simulink model "DePascali4M"  (R2015a)
settings: Solver=ode45  SolverMode=SingleTasking  StartTime=0.0  StopTime=15  RelTol=1e-5
values from neighbouring files (symbols this model uses):
  d1 = 500    [DePascali4Minit.m]    (also in M46Dinit.m)
  d2 = 500    [DePascali4Minit.m]    (also in M46Dinit.m)
  d3 = 500    [DePascali4Minit.m]    (also in M46Dinit.m)
  d4 = 500    [DePascali4Minit.m]    (also in M46Dinit.m)
  delta1 = 200    [DePascali4Minit.m]    (also in M46Dinit.m)
  delta2 = 200    [DePascali4Minit.m]    (also in M46Dinit.m)
  delta3 = 200    [DePascali4Minit.m]    (also in M46Dinit.m)
  delta4 = 200    [DePascali4Minit.m]    (also in M46Dinit.m)
  g = [0;0;9.81]    [DePascali4Minit.m]    (also in M46Dinit.m)
  j0 = 0.5    [DePascali4Minit.m]    (also in M46Dinit.m)
  j1 = 10    [DePascali4Minit.m]    (also in M46Dinit.m = 1)
  j1d = j1    (= 10)    [DePascali4Minit.m]
  j2 = 10    [DePascali4Minit.m]    (also in M46Dinit.m = 1)
  j2d = j2    (= 10)    [DePascali4Minit.m]
  j3 = 10    [DePascali4Minit.m]    (also in M46Dinit.m = 1)
  j3d = j3    (= 10)    [DePascali4Minit.m]
  j4d = j4    (= 10)    [DePascali4Minit.m]
  k1 = 50    [DePascali4Minit.m]    (also in M46Dinit.m = 100)
  k2 = 50    [DePascali4Minit.m]    (also in M46Dinit.m = 100)
  k3 = 50    [DePascali4Minit.m]    (also in M46Dinit.m = 100)
  k4 = 50    [DePascali4Minit.m]    (also in M46Dinit.m = 100)
  kappa1 = 10    [DePascali4Minit.m]    (also in M46Dinit.m = 100)
  kappa2 = 10    [DePascali4Minit.m]    (also in M46Dinit.m = 100)
  kappa3 = 10    [DePascali4Minit.m]    (also in M46Dinit.m = 100)
  kappa4 = 10    [DePascali4Minit.m]    (also in M46Dinit.m = 100)
  m0 = 20    [DePascali4Minit.m]    (also in M46Dinit.m)
  m1 = 100    [DePascali4Minit.m]    (also in M46Dinit.m = 10)
  m1d = m1    (= 100)    [DePascali4Minit.m]
  m2 = 100    [DePascali4Minit.m]    (also in M46Dinit.m = 10)
  m2d = m2    (= 100)    [DePascali4Minit.m]
  m3 = 100    [DePascali4Minit.m]    (also in M46Dinit.m = 10)
  m3d = m3    (= 100)    [DePascali4Minit.m]
  m4 = 100    [DePascali4Minit.m]    (also in M46Dinit.m = 10)
  m4d = m4    (= 100)    [DePascali4Minit.m]
libraries: aerolibutil x7, dspinverses x1
settings Model: CovSFcnEnable=off  Creator=Martin  LastModifiedBy=mangerer
settings DataIOCC: LimitDataPoints=off
settings OptimizationCC: BlockReduction=off  BooleanDataType=off
settings DebuggingCC: SaveWithParameterizedLinksMsg=none  UnderspecifiedInitializationDetection=Classic  MergeDetectMultiDrivingBlocksExec=none  SignalResolutionControl=TryResolveAllWithWarning
settings HardwareCC: TargetUnknown=on

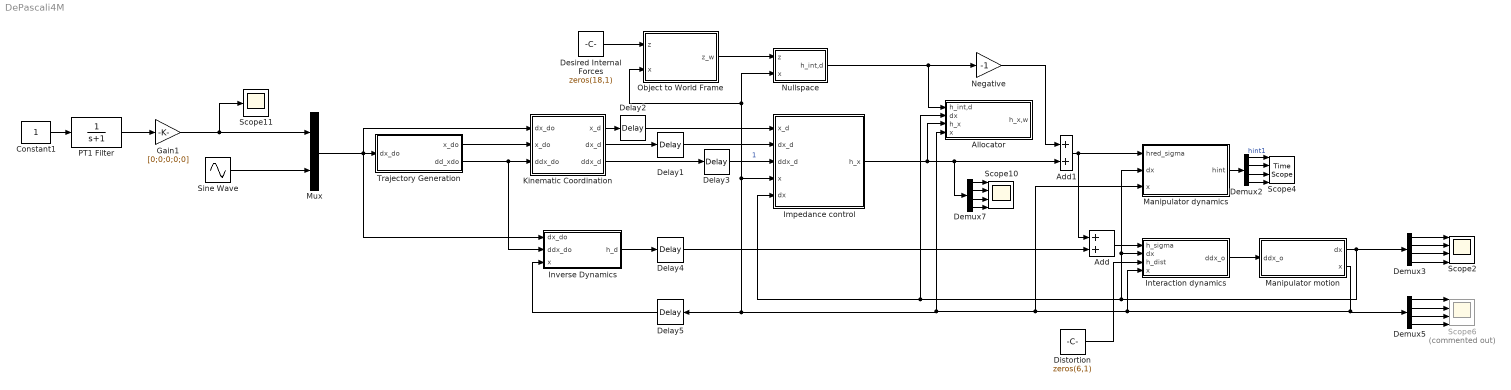
== system DePascali4M ==
  Add : Sum
  Add1 : Sum
  Allocator : Subsystem
  Constant1 : Constant
  Delay1 : TransportDelay  DelayTime=0
  Delay2 : TransportDelay  DelayTime=0  InitialOutput="[1 0 0 1 0 0 0   0 1 0 1 0 0 0    -1 0 0 1 0 0 0     0 -1 0 1 0 0 0]'"
  Delay3 : TransportDelay  DelayTime=0
  Delay4 : TransportDelay  DelayTime=0
  Delay5 : TransportDelay  DelayTime=0  InitialOutput="[1 0 0 1 0 0 0   0 1 0 1 0 0 0    -1 0 0 1 0 0 0     0 -1 0 1 0 0 0]'"
  Demux{2..3,5,7} (4 alike) : Demux
  Desired Internal Forces : Constant  Value=zeros(18,1)
  Distortion : Constant  Value=zeros(6,1)
  Gain1 : Gain  Gain=[0;0;0;0;0]
  Impedance control : Subsystem
  Interaction dynamics : Subsystem
  Inverse Dynamics : Subsystem
  Kinematic Coordination : Subsystem
  Manipulator dynamics : Subsystem
  Manipulator motion : Subsystem
  Mux : Mux  Inputs=2
  Negative : Gain  Gain=-1
  Nullspace : Subsystem
  Object to World Frame : MATLAB Function  TreatAsAtomicUnit=on
  PT1 Filter : TransferFcn  Denominator=[1 1]
  Scope10 : Scope  NumInputPorts=4
      settings: ShowLegends=on  YMin=-1~-5~-5~-5  YMax=1~5~5~5  SaveName=ScopeData18
  Scope11 : Scope
      settings: YMin=0.9984  YMax=1  SaveName=ScopeData26
  Scope2 : Scope  NumInputPorts=4
      settings: ShowLegends=on  YMin=-1.5~-1.5~-1.5~-1.5  YMax=6~5.5~6~5.5  SaveName=ScopeData2
  Scope4 : TimeScope  NumInputPorts=4
  Scope6 : Scope  Commented=on  NumInputPorts=4
      settings: ShowLegends=on  YMin=-25~-25~-25~-25  YMax=200~200~200~200  SaveName=ScopeData11
  Sine Wave : Sin  Frequency=2*pi  SampleTime=0
  Trajectory Generation : Subsystem
  wires:
  Interaction dynamics/1(ddx_o) -> Manipulator motion/1(ddx_o)
  Manipulator dynamics/1(hint) -> Demux2/1
  Demux2/1 -> Scope4/1  "hint1"
  Demux2/2 -> Scope4/2
  Demux2/3 -> Scope4/3
  Demux2/4 -> Scope4/4
  Demux3/1 -> Scope2/1
  Demux3/2 -> Scope2/2
  Demux3/3 -> Scope2/3
  Demux3/4 -> Scope2/4
  Add1/1 -> Manipulator dynamics/1(hred_sigma), Add/1
  Demux5/1 -> Scope6/1
  Demux5/2 -> Scope6/2
  Demux5/3 -> Scope6/3
  Demux5/4 -> Scope6/4
  Object to World Frame/1(z_w) -> Nullspace/1(z)
  Nullspace/1(h_int,d) -> Negative/1, Allocator/1(h_int,d)
  Desired Internal Forces/1 -> Object to World Frame/1(z)
  Demux7/1 -> Scope10/1
  Demux7/2 -> Scope10/2
  Demux7/3 -> Scope10/3
  Demux7/4 -> Scope10/4
  PT1 Filter/1 -> Gain1/1
  Add/1 -> Interaction dynamics/1(h_sigma)
  Gain1/1 -> Scope11/1, Mux/1
  Impedance control/1(h_x) -> Demux7/1, Add1/2, Allocator/3(h_x)
  Manipulator motion/1(dx) -> Demux3/1, Impedance control/5(dx), Allocator/2(dx), Interaction dynamics/2(dx), Manipulator dynamics/2(dx)
  Inverse Dynamics/1(h_d) -> Delay4/1
  Sine Wave/1 -> Mux/2
  Kinematic Coordination/1(x_d) -> Delay2/1
  Kinematic Coordination/2(dx_d) -> Delay1/1
  Kinematic Coordination/3(ddx_d) -> Delay3/1
  Trajectory Generation/2(dd_xdo) -> Kinematic Coordination/3(ddx_do), Inverse Dynamics/2(ddx_do)
  Trajectory Generation/1(x_do) -> Kinematic Coordination/2(x_do)
  Mux/1 -> Kinematic Coordination/1(dx_do), Inverse Dynamics/1(dx_do), Trajectory Generation/1(dx_do)
  Delay2/1 -> Impedance control/1(x_d)
  Delay1/1 -> Impedance control/2(dx_d)
  Delay3/1 -> Impedance control/3(ddx_d)  "1"
  Delay4/1 -> Add/2
  Manipulator motion/2(x) -> Demux5/1, Interaction dynamics/4(x), Manipulator dynamics/3(x), Impedance control/4(x), Object to World Frame/2(x), Nullspace/2(x), Delay5/1, Allocator/4(x)
  Delay5/1 -> Inverse Dynamics/3(x)
  Negative/1 -> Add1/1
  Constant1/1 -> PT1 Filter/1
  Distortion/1 -> Interaction dynamics/3(h_dist)

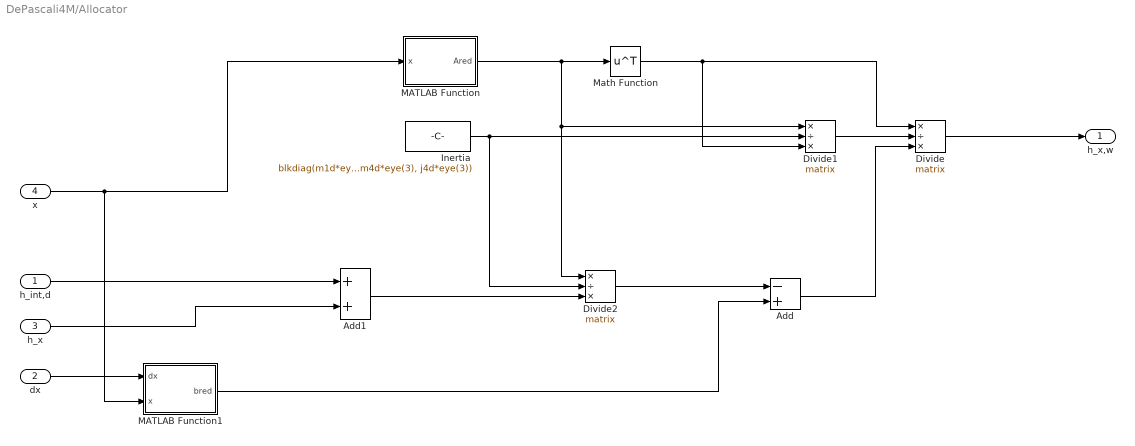
== system DePascali4M/Allocator ==
  h_int,d : Inport
  dx : Inport  Port=2
  h_x : Inport  Port=3
  x : Inport  Port=4
  Add : Sum  Inputs=-+
  Add1 : Sum
  Divide : Product  Inputs=*/*  Multiplication=Matrix(*)
  Divide1 : Product  Inputs=*/*  Multiplication=Matrix(*)
  Divide2 : Product  Inputs=*/*  Multiplication=Matrix(*)
  Inertia : Constant  Value=blkdiag(m1d*eye(3), j1d*eye(3), m2d*eye(3), j2d*eye(3), m3d*eye(3), j3d*eye(3), m4d*eye(3), j4d*eye(3))
  MATLAB Function : MATLAB Function  TreatAsAtomicUnit=on
  MATLAB Function1 : MATLAB Function  TreatAsAtomicUnit=on
  Math Function : Math  Operator=transpose  SaturateOnIntegerOverflow=on
  h_x,w : Outport
  wires:
  dx/1 -> MATLAB Function1/1(dx)
  Divide/1 -> h_x,w/1
  Math Function/1 -> Divide1/3, Divide/1
  MATLAB Function/1(Ared) -> Math Function/1, Divide2/1, Divide1/1
  Divide1/1 -> Divide/2
  Inertia/1 -> Divide1/2, Divide2/2
  MATLAB Function1/1(bred) -> Add/2
  Add/1 -> Divide/3
  Divide2/1 -> Add/1
  Add1/1 -> Divide2/3
  h_int,d/1 -> Add1/1
  h_x/1 -> Add1/2
  x/1 -> MATLAB Function1/2(x), MATLAB Function/1(x)

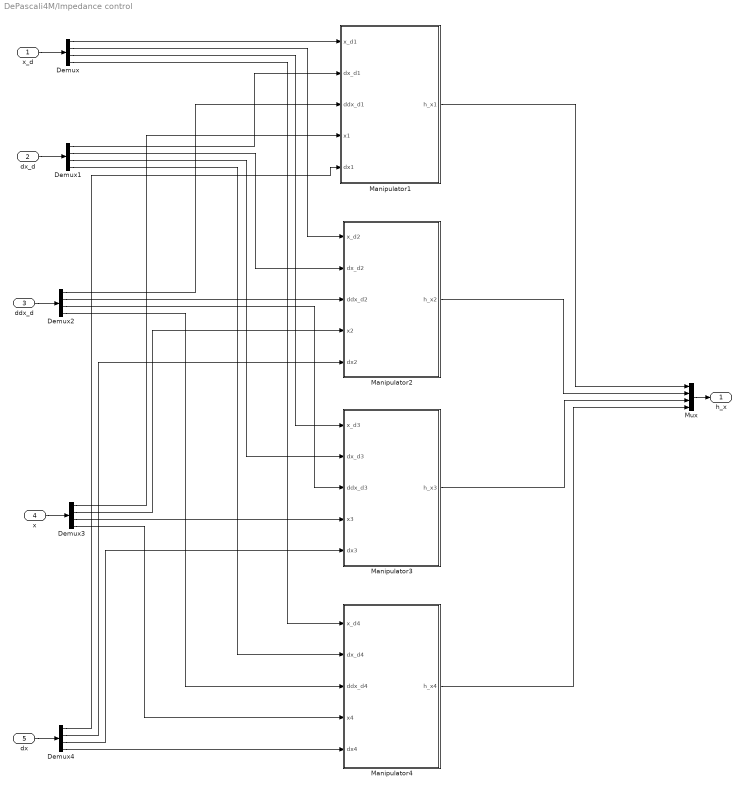
== system DePascali4M/Impedance control ==
  x_d : Inport
  dx_d : Inport  Port=2
  ddx_d : Inport  Port=3
  x : Inport  Port=4
  dx : Inport  Port=5
  Demux{,1..4} (5 alike) : Demux
  Manipulator1 : Subsystem
  Manipulator2 : Subsystem
  Manipulator3 : Subsystem
  Manipulator4 : Subsystem
  Mux : Mux
  h_x : Outport
  wires:
  dx/1 -> Demux4/1
  x/1 -> Demux3/1
  ddx_d/1 -> Demux2/1
  dx_d/1 -> Demux1/1
  x_d/1 -> Demux/1
  Demux/1 -> Manipulator1/1(x_d1)
  Demux/2 -> Manipulator2/1(x_d2)
  Demux/3 -> Manipulator3/1(x_d3)
  Demux/4 -> Manipulator4/1(x_d4)
  Demux1/1 -> Manipulator1/2(dx_d1)
  Demux1/2 -> Manipulator2/2(dx_d2)
  Demux1/3 -> Manipulator3/2(dx_d3)
  Demux1/4 -> Manipulator4/2(dx_d4)
  Demux2/1 -> Manipulator1/3(ddx_d1)
  Demux2/2 -> Manipulator2/3(ddx_d2)
  Demux2/3 -> Manipulator3/3(ddx_d3)
  Demux2/4 -> Manipulator4/3(ddx_d4)
  Demux3/1 -> Manipulator1/4(x1)
  Demux3/2 -> Manipulator2/4(x2)
  Demux3/3 -> Manipulator3/4(x3)
  Demux3/4 -> Manipulator4/4(x4)
  Demux4/4 -> Manipulator4/5(dx4)
  Demux4/3 -> Manipulator3/5(dx3)
  Demux4/2 -> Manipulator2/5(dx2)
  Demux4/1 -> Manipulator1/5(dx1)
  Mux/1 -> h_x/1
  Manipulator1/1(h_x1) -> Mux/1
  Manipulator2/1(h_x2) -> Mux/2
  Manipulator3/1(h_x3) -> Mux/3
  Manipulator4/1(h_x4) -> Mux/4

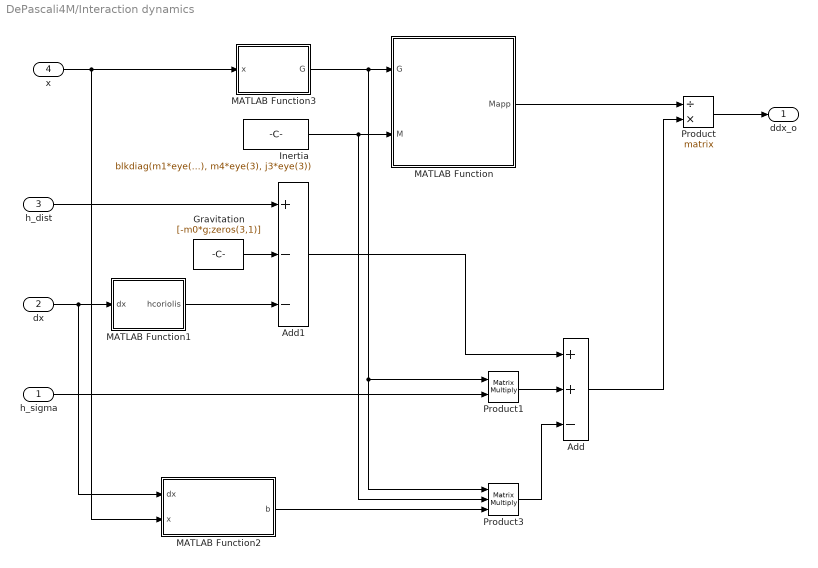
== system DePascali4M/Interaction dynamics ==
  h_sigma : Inport
  dx : Inport  Port=2
  h_dist : Inport  Port=3
  x : Inport  Port=4
  Add : Sum  Inputs=++-
  Add1 : Sum  Inputs=+--
  Gravitation : Constant  Value=[-m0*g;zeros(3,1)]
  Inertia : Constant  Value=blkdiag(m1*eye(3), j1*eye(3), m2*eye(3), j2*eye(3), m3*eye(3), j3*eye(3), m4*eye(3), j3*eye(3))
  MATLAB Function : MATLAB Function  TreatAsAtomicUnit=on
  MATLAB Function1 : MATLAB Function  TreatAsAtomicUnit=on
  MATLAB Function2 : MATLAB Function  TreatAsAtomicUnit=on
  MATLAB Function3 : MATLAB Function  TreatAsAtomicUnit=on
  Product : Product  Inputs=/*  Multiplication=Matrix(*)
  Product1 : Product  Multiplication=Matrix(*)
  Product3 : Product  Inputs=***  Multiplication=Matrix(*)
  ddx_o : Outport
  wires:
  MATLAB Function3/1(G) -> Product1/1, Product3/1, MATLAB Function/1(G)
  Inertia/1 -> Product3/2, MATLAB Function/2(M)
  MATLAB Function/1(Mapp) -> Product/1
  Add/1 -> Product/2
  Product1/1 -> Add/2
  h_sigma/1 -> Product1/2
  Add1/1 -> Add/1
  h_dist/1 -> Add1/1
  Gravitation/1 -> Add1/2
  dx/1 -> MATLAB Function2/1(dx), MATLAB Function1/1(dx)
  MATLAB Function1/1(hcoriolis) -> Add1/3
  Product3/1 -> Add/3
  MATLAB Function2/1(b) -> Product3/3
  Product/1 -> ddx_o/1
  x/1 -> MATLAB Function2/2(x), MATLAB Function3/1(x)

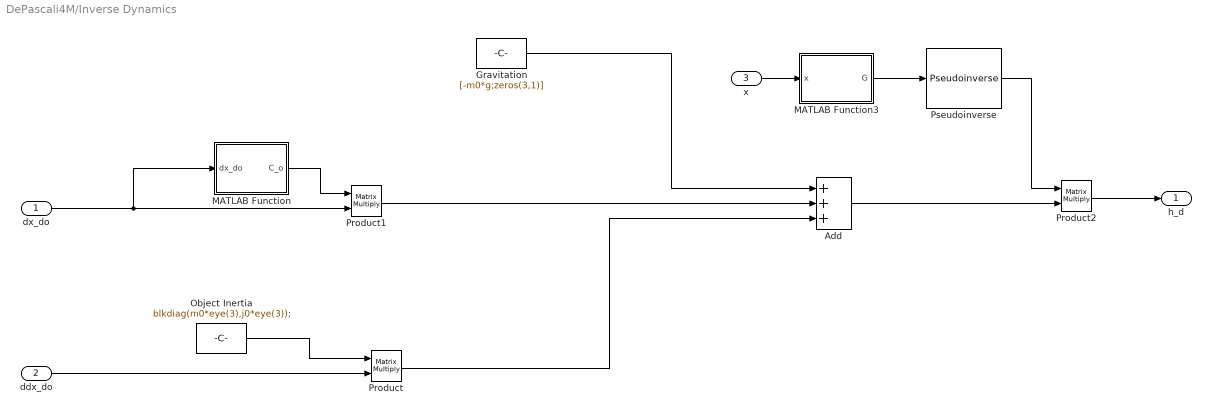
== system DePascali4M/Inverse Dynamics ==
  dx_do : Inport
  ddx_do : Inport  Port=2
  x : Inport  Port=3
  Add : Sum  Inputs=+++
  Gravitation : Constant  Value=[-m0*g;zeros(3,1)]
  MATLAB Function : MATLAB Function  TreatAsAtomicUnit=on
  MATLAB Function3 : MATLAB Function  TreatAsAtomicUnit=on
  Object Inertia : Constant  Value=blkdiag(m0*eye(3),j0*eye(3));
  Product : Product  Multiplication=Matrix(*)
  Product1 : Product  Multiplication=Matrix(*)
  Product2 : Product  Multiplication=Matrix(*)
  Pseudoinverse : dspinverses/Pseudoinverse  wanterr=off
  h_d : Outport
  wires:
  ddx_do/1 -> Product/2
  Object Inertia/1 -> Product/1
  dx_do/1 -> Product1/2, MATLAB Function/1(dx_do)
  MATLAB Function/1(C_o) -> Product1/1
  Product1/1 -> Add/2
  Gravitation/1 -> Add/1
  MATLAB Function3/1(G) -> Pseudoinverse/1
  Pseudoinverse/1 -> Product2/1
  Product2/1 -> h_d/1
  x/1 -> MATLAB Function3/1(x)
  Product/1 -> Add/3
  Add/1 -> Product2/2

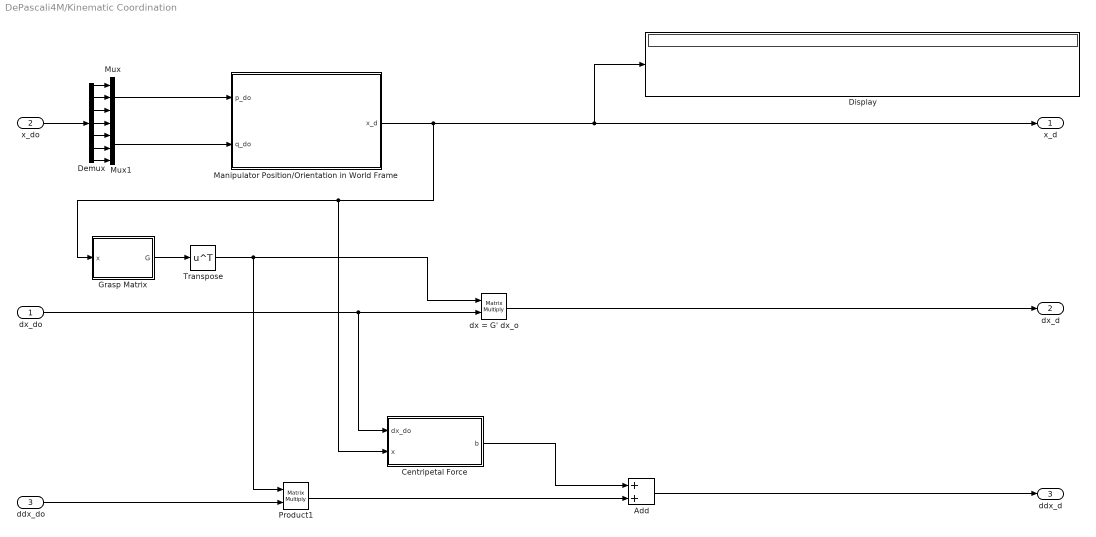
== system DePascali4M/Kinematic Coordination ==
  dx_do : Inport
  x_do : Inport  Port=2
  ddx_do : Inport  Port=3
  Add : Sum
  Centripetal Force : MATLAB Function  TreatAsAtomicUnit=on
  Demux : Demux  Outputs=7
  Display : Display
  Grasp Matrix : MATLAB Function  TreatAsAtomicUnit=on
  Manipulator Position/Orientation in World Frame : MATLAB Function  TreatAsAtomicUnit=on
  Mux : Mux  Inputs=3
  Mux1 : Mux
  Product1 : Product  Multiplication=Matrix(*)
  Transpose : Math  Operator=transpose  SaturateOnIntegerOverflow=on
  dx = G' dx_o : Product  Multiplication=Matrix(*)
  x_d : Outport
  dx_d : Outport  Port=2
  ddx_d : Outport  Port=3
  wires:
  Grasp Matrix/1(G) -> Transpose/1
  Transpose/1 -> Product1/1, dx = G' dx_o/1
  dx_do/1 -> Centripetal Force/1(dx_do), dx = G' dx_o/2
  dx = G' dx_o/1 -> dx_d/1
  x_do/1 -> Demux/1
  Demux/1 -> Mux/1
  Demux/2 -> Mux/2
  Demux/3 -> Mux/3
  Demux/5 -> Mux1/2
  Demux/6 -> Mux1/3
  Demux/7 -> Mux1/4
  Demux/4 -> Mux1/1
  Mux1/1 -> Manipulator Position/Orientation in World Frame/2(q_do)
  Mux/1 -> Manipulator Position/Orientation in World Frame/1(p_do)
  Centripetal Force/1(b) -> Add/1
  ddx_do/1 -> Product1/2
  Product1/1 -> Add/2
  Add/1 -> ddx_d/1
  Manipulator Position/Orientation in World Frame/1(x_d) -> Centripetal Force/2(x), Grasp Matrix/1(x), Display/1, x_d/1

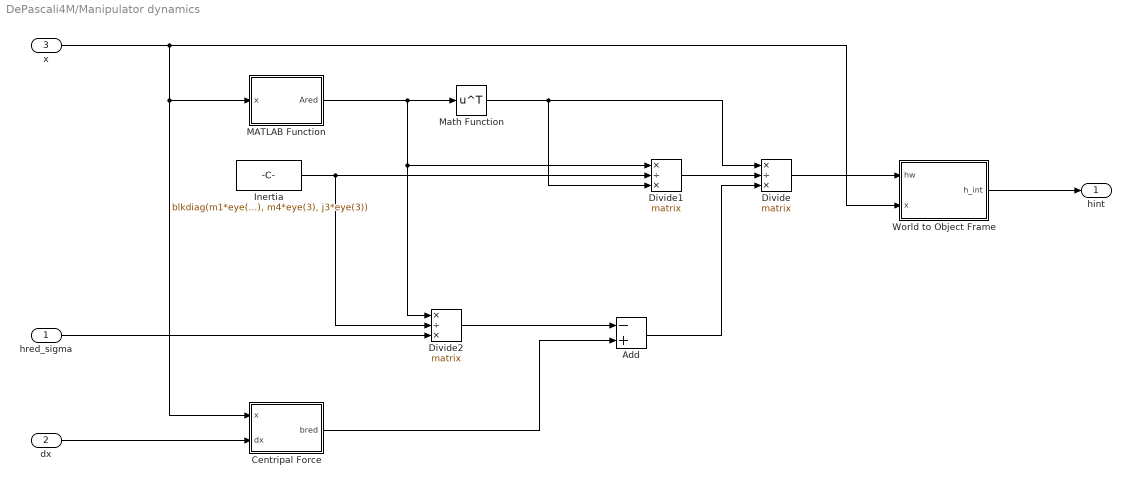
== system DePascali4M/Manipulator dynamics ==
  hred_sigma : Inport
  dx : Inport  Port=2
  x : Inport  Port=3
  Add : Sum  Inputs=-+
  Centripal Force : MATLAB Function  TreatAsAtomicUnit=on
  Divide : Product  Inputs=*/*  Multiplication=Matrix(*)
  Divide1 : Product  Inputs=*/*  Multiplication=Matrix(*)
  Divide2 : Product  Inputs=*/*  Multiplication=Matrix(*)
  Inertia : Constant  Value=blkdiag(m1*eye(3), j1*eye(3), m2*eye(3), j2*eye(3), m3*eye(3), j3*eye(3), m4*eye(3), j3*eye(3))
  MATLAB Function : MATLAB Function  TreatAsAtomicUnit=on
  Math Function : Math  Operator=transpose  SaturateOnIntegerOverflow=on
  World to Object Frame : MATLAB Function  TreatAsAtomicUnit=on
  hint : Outport
  wires:
  Math Function/1 -> Divide1/3, Divide/1
  MATLAB Function/1(Ared) -> Math Function/1, Divide2/1, Divide1/1
  Divide1/1 -> Divide/2
  Inertia/1 -> Divide1/2, Divide2/2
  dx/1 -> Centripal Force/2(dx)
  Add/1 -> Divide/3
  Divide2/1 -> Add/1
  hred_sigma/1 -> Divide2/3
  Divide/1 -> World to Object Frame/1(hw)
  World to Object Frame/1(h_int) -> hint/1
  x/1 -> Centripal Force/1(x), MATLAB Function/1(x), World to Object Frame/2(x)
  Centripal Force/1(bred) -> Add/2

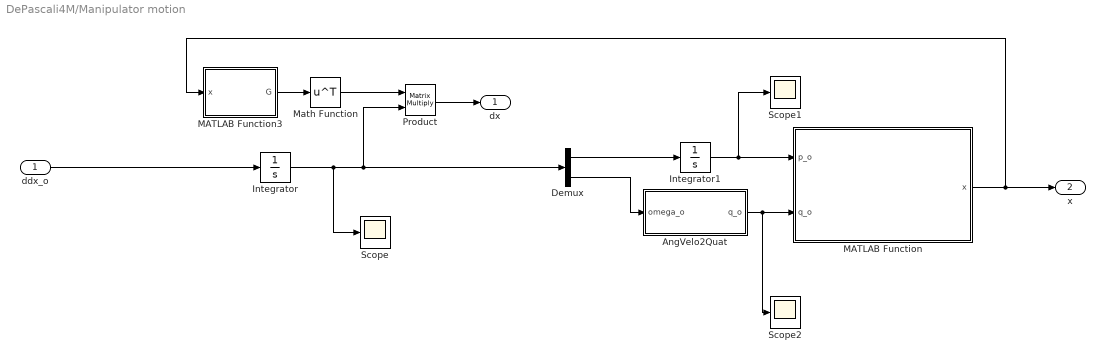
== system DePascali4M/Manipulator motion ==
  ddx_o : Inport
  AngVelo2Quat : Subsystem
  Demux : Demux  Outputs=2
  Integrator : Integrator  InitialCondition=zeros(6,1)
  Integrator1 : Integrator  InitialCondition=[0 0 0]'
  MATLAB Function : MATLAB Function  TreatAsAtomicUnit=on
  MATLAB Function3 : MATLAB Function  TreatAsAtomicUnit=on
  Math Function : Math  Operator=transpose  SaturateOnIntegerOverflow=on
  Product : Product  Multiplication=Matrix(*)
  Scope : Scope
      settings: SaveName=ScopeData14
  Scope1 : Scope
      settings: SaveName=ScopeData15
  Scope2 : Scope
      settings: SaveName=ScopeData23
  dx : Outport
  x : Outport  Port=2
  wires:
  ddx_o/1 -> Integrator/1
  Integrator/1 -> Scope/1, Product/2, Demux/1
  MATLAB Function3/1(G) -> Math Function/1
  Math Function/1 -> Product/1
  Product/1 -> dx/1
  Demux/2 -> AngVelo2Quat/1(omega_o)
  Demux/1 -> Integrator1/1
  AngVelo2Quat/1(q_o) -> Scope2/1, MATLAB Function/2(q_o)
  Integrator1/1 -> Scope1/1, MATLAB Function/1(p_o)
  MATLAB Function/1(x) -> MATLAB Function3/1(x), x/1

== system DePascali4M/Nullspace ==
  z : Inport
  x : Inport  Port=2
  MATLAB Function : MATLAB Function  TreatAsAtomicUnit=on
  Math Function : Math  Operator=transpose  SaturateOnIntegerOverflow=on
  Product : Product  Multiplication=Matrix(*)
  h_int,d : Outport
  wires:
  MATLAB Function/1(Ared) -> Math Function/1
  Math Function/1 -> Product/1
  z/1 -> Product/2
  Product/1 -> h_int,d/1
  x/1 -> MATLAB Function/1(x)

== system DePascali4M/Trajectory Generation ==
  dx_do : Inport
  Angular Velocity to Quaternion Orientation : Subsystem
  Demux : Demux  Outputs=2
  Derivative : Derivative
  Integrator : Integrator  InitialCondition=zeros(3,1)
  Mux : Mux  Inputs=2
  Scope : Scope
      settings: YMin=-12.5  YMax=12.5  SaveName=ScopeData25
  x_do : Outport
  dd_xdo : Outport  Port=2
  wires:
  dx_do/1 -> Derivative/1, Demux/1
  Demux/2 -> Angular Velocity to Quaternion Orientation/1(omega_do)
  Demux/1 -> Integrator/1
  Angular Velocity to Quaternion Orientation/1(q_do) -> Mux/2
  Integrator/1 -> Mux/1
  Mux/1 -> x_do/1
  Derivative/1 -> Scope/1, dd_xdo/1

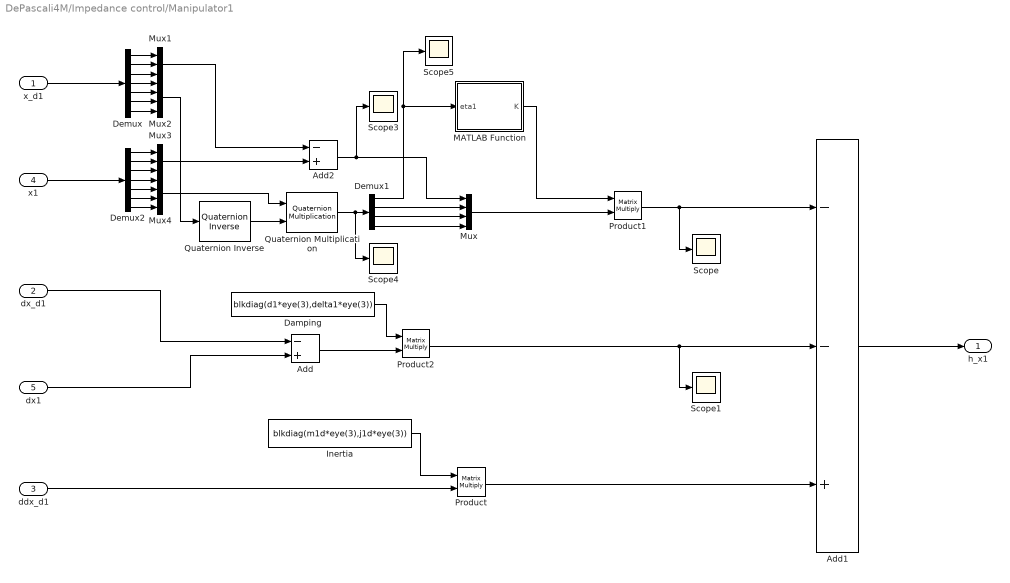
== system DePascali4M/Impedance control/Manipulator1 ==
  x_d1 : Inport
  dx_d1 : Inport  Port=2
  ddx_d1 : Inport  Port=3
  x1 : Inport  Port=4
  dx1 : Inport  Port=5
  Add : Sum  Inputs=-+
  Add1 : Sum  Inputs=--+
  Add2 : Sum  Inputs=-+
  Damping : Constant  Value=blkdiag(d1*eye(3),delta1*eye(3))
  Demux : Demux  Outputs=7
  Demux1 : Demux
  Demux2 : Demux  Outputs=7
  Inertia : Constant  Value=blkdiag(m1d*eye(3),j1d*eye(3))
  MATLAB Function : MATLAB Function  TreatAsAtomicUnit=on
  Mux : Mux
  Mux1 : Mux  Inputs=3
  Mux2 : Mux
  Mux3 : Mux  Inputs=3
  Mux4 : Mux
  Product : Product  Multiplication=Matrix(*)
  Product1 : Product  Multiplication=Matrix(*)
  Product2 : Product  Multiplication=Matrix(*)
  Quaternion Inverse : aerolibutil/Quaternion Inverse
  Quaternion Multiplication : aerolibutil/Quaternion Multiplication
  Scope{,1,3..5} (5 alike) : Scope
      Scope settings: TimeRange=200  YMin=-50  YMax=125  SaveName=ScopeData13
      Scope1 settings: TimeRange=200  YMin=-50  YMax=125  SaveName=ScopeData19
      Scope3 settings: ShowLegends=on  TimeRange=200  YMin=-50  YMax=125  SaveName=ScopeData21
      Scope4 settings: ShowLegends=on  TimeRange=50  YMin=-0.05  YMax=1  SaveName=ScopeData22
      Scope5 settings: ShowLegends=on  TimeRange=200  YMin=-50  YMax=125  SaveName=ScopeData24
  h_x1 : Outport
  wires:
  Add/1 -> Product2/2
  Damping/1 -> Product2/1
  dx_d1/1 -> Add/1
  dx1/1 -> Add/2
  MATLAB Function/1(K) -> Product1/1
  Demux1/1 -> MATLAB Function/1(eta1), Scope5/1
  Add2/1 -> Scope3/1, Mux/1
  Demux1/2 -> Mux/2
  Demux1/3 -> Mux/3
  Demux1/4 -> Mux/4
  x1/1 -> Demux2/1
  x_d1/1 -> Demux/1
  Demux/2 -> Mux1/2
  Demux/1 -> Mux1/1
  Demux/3 -> Mux1/3
  Demux/4 -> Mux2/1
  Demux/5 -> Mux2/2
  Demux/6 -> Mux2/3
  Demux/7 -> Mux2/4
  Demux2/2 -> Mux3/2
  Demux2/1 -> Mux3/1
  Demux2/3 -> Mux3/3
  Demux2/4 -> Mux4/1
  Demux2/5 -> Mux4/2
  Demux2/6 -> Mux4/3
  Demux2/7 -> Mux4/4
  Mux1/1 -> Add2/1
  Mux3/1 -> Add2/2
  Quaternion Multiplication/1 -> Scope4/1, Demux1/1
  Mux/1 -> Product1/2
  Inertia/1 -> Product/1
  Add1/1 -> h_x1/1
  Product1/1 -> Scope/1, Add1/1
  Product2/1 -> Scope1/1, Add1/2
  Product/1 -> Add1/3
  Quaternion Inverse/1 -> Quaternion Multiplication/2
  Mux4/1 -> Quaternion Multiplication/1
  Mux2/1 -> Quaternion Inverse/1
  ddx_d1/1 -> Product/2

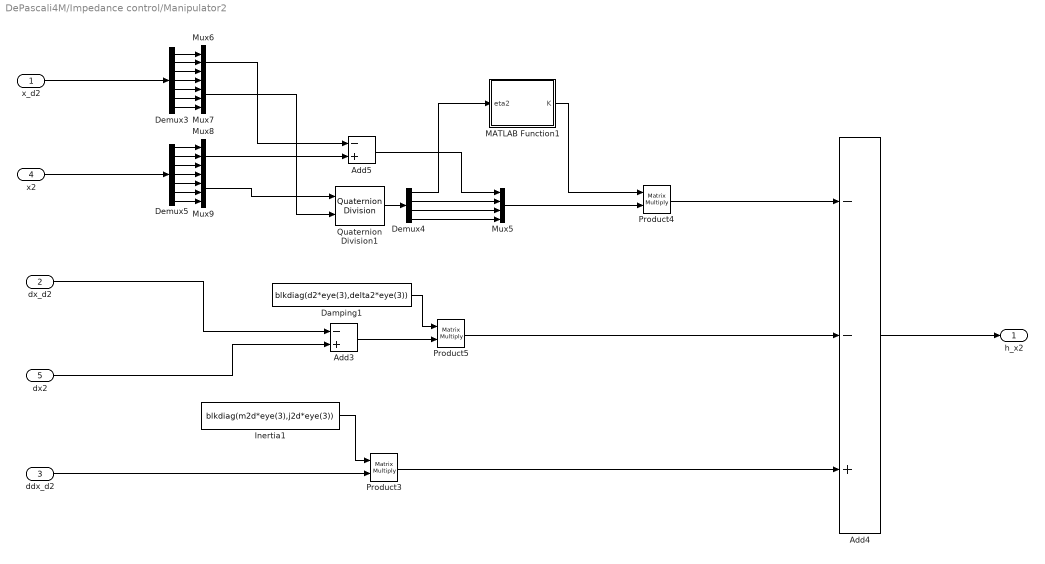
== system DePascali4M/Impedance control/Manipulator2 ==
  x_d2 : Inport
  dx_d2 : Inport  Port=2
  ddx_d2 : Inport  Port=3
  x2 : Inport  Port=4
  dx2 : Inport  Port=5
  Add3 : Sum  Inputs=-+
  Add4 : Sum  Inputs=--+
  Add5 : Sum  Inputs=-+
  Damping1 : Constant  Value=blkdiag(d2*eye(3),delta2*eye(3))
  Demux3 : Demux  Outputs=7
  Demux4 : Demux
  Demux5 : Demux  Outputs=7
  Inertia1 : Constant  Value=blkdiag(m2d*eye(3),j2d*eye(3))
  MATLAB Function1 : MATLAB Function  TreatAsAtomicUnit=on
  Mux5 : Mux
  Mux6 : Mux  Inputs=3
  Mux7 : Mux
  Mux8 : Mux  Inputs=3
  Mux9 : Mux
  Product3 : Product  Multiplication=Matrix(*)
  Product4 : Product  Multiplication=Matrix(*)
  Product5 : Product  Multiplication=Matrix(*)
  Quaternion Division1 : aerolibutil/Quaternion Division
  h_x2 : Outport
  wires:
  Add3/1 -> Product5/2
  Damping1/1 -> Product5/1
  dx_d2/1 -> Add3/1
  dx2/1 -> Add3/2
  MATLAB Function1/1(K) -> Product4/1
  Demux4/1 -> MATLAB Function1/1(eta2)
  Add5/1 -> Mux5/1
  Demux4/2 -> Mux5/2
  Demux4/3 -> Mux5/3
  Demux4/4 -> Mux5/4
  x2/1 -> Demux5/1
  x_d2/1 -> Demux3/1
  Demux3/2 -> Mux6/2
  Demux3/1 -> Mux6/1
  Demux3/3 -> Mux6/3
  Demux3/4 -> Mux7/1
  Demux3/5 -> Mux7/2
  Demux3/6 -> Mux7/3
  Demux3/7 -> Mux7/4
  Demux5/2 -> Mux8/2
  Demux5/1 -> Mux8/1
  Demux5/3 -> Mux8/3
  Demux5/4 -> Mux9/1
  Demux5/5 -> Mux9/2
  Demux5/6 -> Mux9/3
  Demux5/7 -> Mux9/4
  Mux6/1 -> Add5/1
  Mux8/1 -> Add5/2
  Quaternion Division1/1 -> Demux4/1
  Mux5/1 -> Product4/2
  Inertia1/1 -> Product3/1
  Add4/1 -> h_x2/1
  Product4/1 -> Add4/1
  Product5/1 -> Add4/2
  Product3/1 -> Add4/3
  Mux7/1 -> Quaternion Division1/2
  Mux9/1 -> Quaternion Division1/1
  ddx_d2/1 -> Product3/2

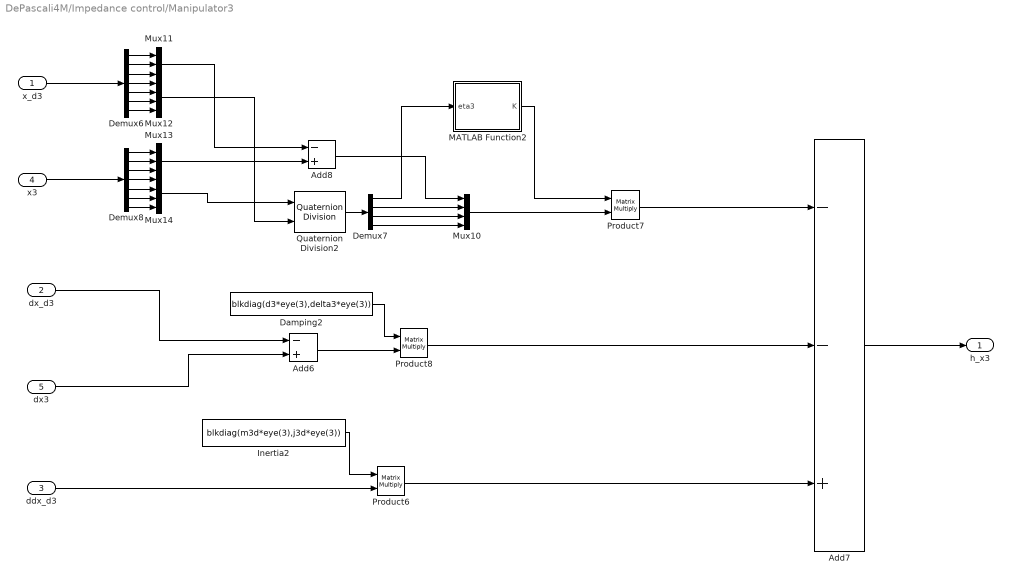
== system DePascali4M/Impedance control/Manipulator3 ==
  x_d3 : Inport
  dx_d3 : Inport  Port=2
  ddx_d3 : Inport  Port=3
  x3 : Inport  Port=4
  dx3 : Inport  Port=5
  Add6 : Sum  Inputs=-+
  Add7 : Sum  Inputs=--+
  Add8 : Sum  Inputs=-+
  Damping2 : Constant  Value=blkdiag(d3*eye(3),delta3*eye(3))
  Demux6 : Demux  Outputs=7
  Demux7 : Demux
  Demux8 : Demux  Outputs=7
  Inertia2 : Constant  Value=blkdiag(m3d*eye(3),j3d*eye(3))
  MATLAB Function2 : MATLAB Function  TreatAsAtomicUnit=on
  Mux10 : Mux
  Mux11 : Mux  Inputs=3
  Mux12 : Mux
  Mux13 : Mux  Inputs=3
  Mux14 : Mux
  Product6 : Product  Multiplication=Matrix(*)
  Product7 : Product  Multiplication=Matrix(*)
  Product8 : Product  Multiplication=Matrix(*)
  Quaternion Division2 : aerolibutil/Quaternion Division
  h_x3 : Outport
  wires:
  Add6/1 -> Product8/2
  Damping2/1 -> Product8/1
  dx_d3/1 -> Add6/1
  dx3/1 -> Add6/2
  MATLAB Function2/1(K) -> Product7/1
  Demux7/1 -> MATLAB Function2/1(eta3)
  Add8/1 -> Mux10/1
  Demux7/2 -> Mux10/2
  Demux7/3 -> Mux10/3
  Demux7/4 -> Mux10/4
  x3/1 -> Demux8/1
  x_d3/1 -> Demux6/1
  Demux6/2 -> Mux11/2
  Demux6/1 -> Mux11/1
  Demux6/3 -> Mux11/3
  Demux6/4 -> Mux12/1
  Demux6/5 -> Mux12/2
  Demux6/6 -> Mux12/3
  Demux6/7 -> Mux12/4
  Demux8/2 -> Mux13/2
  Demux8/1 -> Mux13/1
  Demux8/3 -> Mux13/3
  Demux8/4 -> Mux14/1
  Demux8/5 -> Mux14/2
  Demux8/6 -> Mux14/3
  Demux8/7 -> Mux14/4
  Mux11/1 -> Add8/1
  Mux13/1 -> Add8/2
  Quaternion Division2/1 -> Demux7/1
  Mux10/1 -> Product7/2
  Inertia2/1 -> Product6/1
  Add7/1 -> h_x3/1
  Product7/1 -> Add7/1
  Product8/1 -> Add7/2
  Product6/1 -> Add7/3
  Mux12/1 -> Quaternion Division2/2
  Mux14/1 -> Quaternion Division2/1
  ddx_d3/1 -> Product6/2

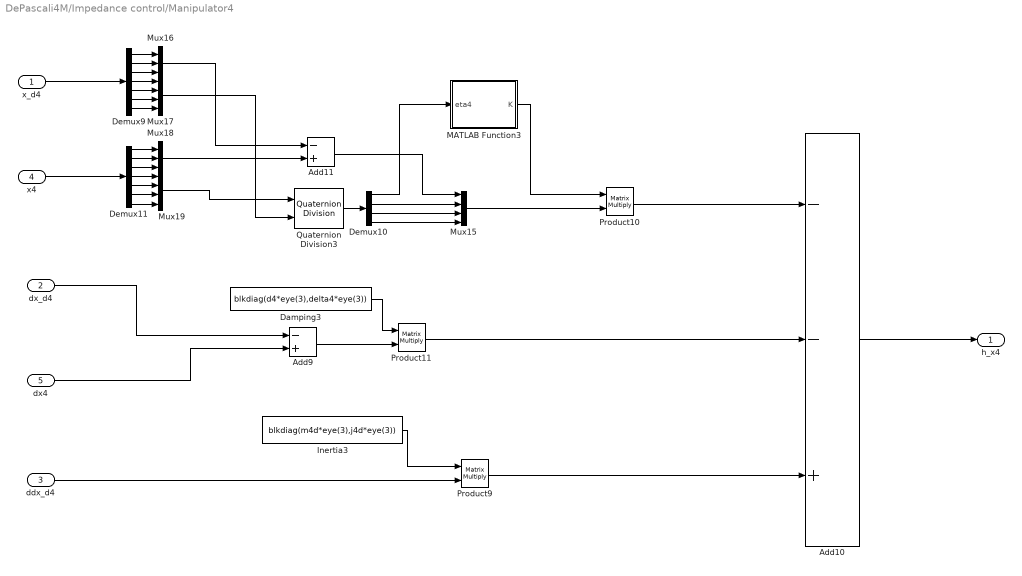
== system DePascali4M/Impedance control/Manipulator4 ==
  x_d4 : Inport
  dx_d4 : Inport  Port=2
  ddx_d4 : Inport  Port=3
  x4 : Inport  Port=4
  dx4 : Inport  Port=5
  Add10 : Sum  Inputs=--+
  Add11 : Sum  Inputs=-+
  Add9 : Sum  Inputs=-+
  Damping3 : Constant  Value=blkdiag(d4*eye(3),delta4*eye(3))
  Demux10 : Demux
  Demux11 : Demux  Outputs=7
  Demux9 : Demux  Outputs=7
  Inertia3 : Constant  Value=blkdiag(m4d*eye(3),j4d*eye(3))
  MATLAB Function3 : MATLAB Function  TreatAsAtomicUnit=on
  Mux15 : Mux
  Mux16 : Mux  Inputs=3
  Mux17 : Mux
  Mux18 : Mux  Inputs=3
  Mux19 : Mux
  Product10 : Product  Multiplication=Matrix(*)
  Product11 : Product  Multiplication=Matrix(*)
  Product9 : Product  Multiplication=Matrix(*)
  Quaternion Division3 : aerolibutil/Quaternion Division
  h_x4 : Outport
  wires:
  Add9/1 -> Product11/2
  Damping3/1 -> Product11/1
  dx_d4/1 -> Add9/1
  dx4/1 -> Add9/2
  MATLAB Function3/1(K) -> Product10/1
  Demux10/1 -> MATLAB Function3/1(eta4)
  Add11/1 -> Mux15/1
  Demux10/2 -> Mux15/2
  Demux10/3 -> Mux15/3
  Demux10/4 -> Mux15/4
  x4/1 -> Demux11/1
  x_d4/1 -> Demux9/1
  Demux9/2 -> Mux16/2
  Demux9/1 -> Mux16/1
  Demux9/3 -> Mux16/3
  Demux9/4 -> Mux17/1
  Demux9/5 -> Mux17/2
  Demux9/6 -> Mux17/3
  Demux9/7 -> Mux17/4
  Demux11/2 -> Mux18/2
  Demux11/1 -> Mux18/1
  Demux11/3 -> Mux18/3
  Demux11/4 -> Mux19/1
  Demux11/5 -> Mux19/2
  Demux11/6 -> Mux19/3
  Demux11/7 -> Mux19/4
  Mux16/1 -> Add11/1
  Mux18/1 -> Add11/2
  Quaternion Division3/1 -> Demux10/1
  Mux15/1 -> Product10/2
  Inertia3/1 -> Product9/1
  Add10/1 -> h_x4/1
  Product10/1 -> Add10/1
  Product11/1 -> Add10/2
  Product9/1 -> Add10/3
  Mux17/1 -> Quaternion Division3/2
  Mux19/1 -> Quaternion Division3/1
  ddx_d4/1 -> Product9/2

== system DePascali4M/Manipulator motion/AngVelo2Quat ==
  omega_o : Inport
  Constant : Constant  Value=0
  Gain : Gain  Gain=0.5
  Integrator : Integrator  InitialCondition=[1; 0; 0; 0]
  Mux : Mux  Inputs=2
  Quaternion Multiplication : aerolibutil/Quaternion Multiplication
  Scope : Scope
      settings: ShowLegends=on  SaveName=ScopeData9
  q_o : Outport
  wires:
  omega_o/1 -> Gain/1
  Gain/1 -> Mux/2
  Constant/1 -> Mux/1
  Quaternion Multiplication/1 -> Integrator/1
  Integrator/1 -> Quaternion Multiplication/2, Scope/1, q_o/1
  Mux/1 -> Quaternion Multiplication/1

== system DePascali4M/Trajectory Generation/Angular Velocity to Quaternion Orientation ==
  omega_do : Inport
  Constant : Constant  Value=0
  Gain : Gain  Gain=0.5
  Integrator : Integrator  InitialCondition=[1; 0; 0; 0]
  Mux : Mux  Inputs=2
  Quaternion Multiplication : aerolibutil/Quaternion Multiplication
  Scope : Scope
      settings: ShowLegends=on  SaveName=ScopeData9
  q_do : Outport
  wires:
  omega_do/1 -> Gain/1
  Gain/1 -> Mux/2
  Constant/1 -> Mux/1
  Quaternion Multiplication/1 -> Integrator/1
  Integrator/1 -> Quaternion Multiplication/2, Scope/1, q_do/1
  Mux/1 -> Quaternion Multiplication/1

== matlab function DePascali4M/Kinematic Coordination/Grasp Matrix ==
  data: r parameter; G output; x input
function G = GraspMatrix(r,x)
G = [eye(3) zeros(3) eye(3) zeros(3) eye(3) zeros(3) eye(3) zeros(3);
    skew_sm(quatrot(x(4:7),r(1:3))) eye(3) skew_sm(quatrot(x(4:7),r(4:6))) eye(3) skew_sm(quatrot(x(4:7),r(7:9))) eye(3) skew_sm(quatrot(x(4:7),r(10:12))) eye(3)];

== matlab function DePascali4M/Kinematic Coordination/Manipulator Position//Orientation in World Frame ==
  data: p_do input; q_do input; x_d output; r parameter
function x_d = manipulatorpose(p_do,q_do,r)
pq_d1 = quatmultiply(quatconj(q_do'),quatmultiply([0 r(1:3)'],q_do'))';
pq_d2 = quatmultiply(quatconj(q_do'),quatmultiply([0 r(4:6)'],q_do'))';
pq_d3 = quatmultiply(quatconj(q_do'),quatmultiply([0 r(7:9)'],q_do'))';
pq_d4 = quatmultiply(quatconj(q_do'),quatmultiply([0 r(10:12)'],q_do'))';


x_d = [p_do + pq_d1(2:4);
        q_do;
        p_do + pq_d2(2:4);
        q_do;
        p_do + pq_d3(2:4);
        q_do;
        p_do + pq_d4(2:4);
        q_do ];

== matlab function DePascali4M/Kinematic Coordination/Centripetal Force ==
  data: dx_do input; b output; r parameter; x input
function b = centripetalforce(dx_do,r,x)
b = [skew_sm(dx_do(4:6))*skew_sm(dx_do(4:6))*quatrot(x(4:7),r(1:3));
     zeros(3,1);
     skew_sm(dx_do(4:6))*skew_sm(dx_do(4:6))*quatrot(x(4:7),r(4:6));
     zeros(3,1);
     skew_sm(dx_do(4:6))*skew_sm(dx_do(4:6))*quatrot(x(4:7),r(7:9));
     zeros(3,1);
     skew_sm(dx_do(4:6))*skew_sm(dx_do(4:6))*quatrot(x(4:7),r(10:12));
     zeros(3,1)];

== matlab function DePascali4M/Inverse Dynamics/MATLAB Function ==
  data: dx_do input; C_o output; j0 parameter
function C_o = Coriolis(dx_do,j0)
C_o = [zeros(3,6);
        zeros(3) j0*skew_sm(dx_do(4:6))];

== matlab function DePascali4M/Inverse Dynamics/MATLAB Function3 ==
  data: r parameter; G output; x input
function G = GraspMatrix(r,x)
G = [eye(3) zeros(3) eye(3) zeros(3) eye(3) zeros(3) eye(3) zeros(3);
    skew_sm(quatrot(x(4:7),r(1:3))) eye(3) skew_sm(quatrot(x(4:7),r(4:6))) eye(3) skew_sm(quatrot(x(4:7),r(7:9))) eye(3) skew_sm(quatrot(x(4:7),r(10:12))) eye(3)];

== matlab function DePascali4M/Impedance control/Manipulator1/MATLAB Function ==
  data: eta1 input; K output; k1 parameter; kappa1 parameter
function K = stiffness(eta1,k1,kappa1)
K = blkdiag(k1*eye(3),2*eta1*kappa1*eye(3));

== matlab function DePascali4M/Impedance control/Manipulator2/MATLAB Function1 ==
  data: eta2 input; K output; k2 parameter; kappa2 parameter
function K = stiffness(eta2,k2,kappa2)
K = blkdiag(k2*eye(3),2*eta2*kappa2*eye(3));

== matlab function DePascali4M/Impedance control/Manipulator3/MATLAB Function2 ==
  data: eta3 input; K output; k3 parameter; kappa3 parameter
function K = stiffness(eta3,k3,kappa3)
K = blkdiag(k3*eye(3),2*eta3*kappa3*eye(3));

== matlab function DePascali4M/Impedance control/Manipulator4/MATLAB Function3 ==
  data: eta4 input; K output; k4 parameter; kappa4 parameter
function K = stiffness(eta4,k4,kappa4)
K = blkdiag(k4*eye(3),2*eta4*kappa4*eye(3));

== matlab function DePascali4M/Manipulator dynamics/MATLAB Function ==
  data: r parameter; Ared output; x input
function Ared = ReducedConstraintMAtrix(r,x)
Ared = [-eye(3) skew_sm(quatrot(x(4:7),r(4:6)-r(1:3))) eye(3) zeros(3,15);
        zeros(3) -eye(3) zeros(3) eye(3) zeros(3,12);
        -eye(3) skew_sm(quatrot(x(4:7),r(7:9)-r(1:3))) zeros(3,6) eye(3) zeros(3,9);
        zeros(3) -eye(3) zeros(3,9) eye(3) zeros(3,6);
        -eye(3) skew_sm(quatrot(x(4:7),r(10:12)-r(1:3))) zeros(3,12) eye(3) zeros(3);
        zeros(3) -eye(3) zeros(3,15) eye(3)];

== matlab function DePascali4M/Manipulator dynamics/Centripal Force ==
  data: r parameter; x input; bred output; dx input
function bred = ReducedCentripetalvector(r,x,dx)
bred = [skew_sm(dx(4:6))*skew_sm(dx(4:6))*quatrot(x(4:7),(r(4:6)-r(1:3)));
        zeros(3,1);
        skew_sm(dx(4:6))*skew_sm(dx(4:6))*quatrot(x(4:7),(r(7:9)-r(1:3)));
        zeros(3,1);
        skew_sm(dx(4:6))*skew_sm(dx(4:6))*quatrot(x(4:7),(r(10:12)-r(1:3)));
        zeros(3,1)];

== matlab function DePascali4M/Interaction dynamics/MATLAB Function ==
  data: G input; Mapp output; M input; m0 parameter; j0 parameter
function Mapp = ApparentInertia(G,M,m0,j0)
Mapp = blkdiag(m0*eye(3),j0*eye(3)) + G*M*G';

== matlab function DePascali4M/Interaction dynamics/MATLAB Function3 ==
  data: r parameter; G output; x input
function G = GraspMatrix(r,x)
G = [eye(3) zeros(3) eye(3) zeros(3) eye(3) zeros(3) eye(3) zeros(3);
    skew_sm(quatrot(x(4:7),r(1:3))) eye(3) skew_sm(quatrot(x(4:7),r(4:6))) eye(3) skew_sm(quatrot(x(4:7),r(7:9))) eye(3) skew_sm(quatrot(x(4:7),r(10:12))) eye(3)];

== matlab function DePascali4M/Interaction dynamics/MATLAB Function1 ==
  data: dx input; hcoriolis output; j0 parameter
function hcoriolis = CoriolisForce(dx,j0)
hcoriolis = [zeros(3,1);
        j0*skew_sm(dx(4:6))*dx(4:6)];

== matlab function DePascali4M/Interaction dynamics/MATLAB Function2 ==
  data: dx input; b output; r parameter; x input
function b = centripetalforce(dx,r,x)
b = [skew_sm(dx(4:6))*skew_sm(dx(4:6))*quatrot(x(4:7),r(1:3));
     zeros(3,1);
     skew_sm(dx(4:6))*skew_sm(dx(4:6))*quatrot(x(4:7),r(4:6));
     zeros(3,1);
     skew_sm(dx(4:6))*skew_sm(dx(4:6))*quatrot(x(4:7),r(7:9));
     zeros(3,1);
     skew_sm(dx(4:6))*skew_sm(dx(4:6))*quatrot(x(4:7),r(10:12));
     zeros(3,1)];

== matlab function DePascali4M/Manipulator motion/MATLAB Function3 ==
  data: r parameter; G output; x input
function G = GraspMatrix(r,x)
G = [eye(3) zeros(3) eye(3) zeros(3) eye(3) zeros(3) eye(3) zeros(3);
    skew_sm(quatrot(x(4:7),r(1:3))) eye(3) skew_sm(quatrot(x(4:7),r(4:6))) eye(3) skew_sm(quatrot(x(4:7),r(7:9))) eye(3) skew_sm(quatrot(x(4:7),r(10:12))) eye(3)];

== matlab function DePascali4M/Manipulator motion/MATLAB Function ==
  data: p_o input; q_o input; x output; r parameter
function x = manipulatorpose(p_o,q_o,r)
pq1 = quatmultiply(quatconj(q_o'),quatmultiply([0 r(1:3)'],q_o'))';
pq2 = quatmultiply(quatconj(q_o'),quatmultiply([0 r(4:6)'],q_o'))';
pq3 = quatmultiply(quatconj(q_o'),quatmultiply([0 r(7:9)'],q_o'))';
pq4 = quatmultiply(quatconj(q_o'),quatmultiply([0 r(10:12)'],q_o'))';


x = [p_o + pq1(2:4);
        q_o;
        p_o + pq2(2:4);
        q_o;
        p_o + pq3(2:4);
        q_o;
        p_o + pq4(2:4);
        q_o ];

== matlab function DePascali4M/Nullspace/MATLAB Function ==
  data: r parameter; Ared output; x input
function Ared = ReducedConstraintMAtrix(r,x)
Ared = [-eye(3) skew_sm(quatrot(x(4:7),r(4:6)-r(1:3))) eye(3) zeros(3,15);
        zeros(3) -eye(3) zeros(3) eye(3) zeros(3,12);
        -eye(3) skew_sm(quatrot(x(4:7),r(7:9)-r(1:3))) zeros(3,6) eye(3) zeros(3,9);
        zeros(3) -eye(3) zeros(3,9) eye(3) zeros(3,6);
        -eye(3) skew_sm(quatrot(x(4:7),r(10:12)-r(1:3))) zeros(3,12) eye(3) zeros(3);
        zeros(3) -eye(3) zeros(3,15) eye(3)];

== matlab function DePascali4M/Allocator/MATLAB Function1 ==
  data: r parameter; bred output; dx input; x input
function bred = ReducedCentripetalvector(r,dx,x)
bred = [skew_sm(dx(4:6))*skew_sm(dx(4:6))*quatrot(x(4:7),r(4:6)-r(1:3));
    zeros(3,1);
    skew_sm(dx(4:6))*skew_sm(dx(4:6))*quatrot(x(4:7),r(7:9)-r(1:3));
    zeros(3,1);
    skew_sm(dx(4:6))*skew_sm(dx(4:6))*quatrot(x(4:7),r(10:12)-r(1:3));
    zeros(3,1)];

== matlab function DePascali4M/Allocator/MATLAB Function ==
  data: r parameter; Ared output; x input
function Ared = ReducedConstraintMAtrix(r,x)
Ared = [-eye(3) skew_sm(quatrot(x(4:7),r(4:6)-r(1:3))) eye(3) zeros(3,15);
        zeros(3) -eye(3) zeros(3) eye(3) zeros(3,12);
        -eye(3) skew_sm(quatrot(x(4:7),r(7:9)-r(1:3))) zeros(3,6) eye(3) zeros(3,9);
        zeros(3) -eye(3) zeros(3,9) eye(3) zeros(3,6);
        -eye(3) skew_sm(quatrot(x(4:7),r(10:12)-r(1:3))) zeros(3,12) eye(3) zeros(3);
        zeros(3) -eye(3) zeros(3,15) eye(3)];

== matlab function DePascali4M/Object to World Frame ==
  data: z input; x input; z_w output
function z_w = object2inertialFrame(z,x)
zwt1 = quatmultiply(quatconj(x(4:7)'),quatmultiply([0 z(1:3)'],x(4:7)'))';
zwt2 = quatmultiply(quatconj(x(4:7)'),quatmultiply([0 z(7:9)'],x(4:7)'))';
zwt3 = quatmultiply(quatconj(x(4:7)'),quatmultiply([0 z(13:15)'],x(4:7)'))';
zwr1 = quatmultiply(quatconj(x(4:7)'),quatmultiply([0 z(4:6)'],x(4:7)'))';
zwr2 = quatmultiply(quatconj(x(4:7)'),quatmultiply([0 z(10:12)'],x(4:7)'))';
zwr3 = quatmultiply(quatconj(x(4:7)'),quatmultiply([0 z(16:18)'],x(4:7)'))';


z_w = [zwt1(2:4);
        zwr1(2:4);
        zwt2(2:4);
        zwr2(2:4);
        zwt3(2:4);
        zwr3(2:4)];

== matlab function DePascali4M/Manipulator dynamics/World to Object Frame ==
  data: hw input; x input; h_int output
function h_int = inertial2objectFrame(hw,x)
hint1  = quatmultiply(x(4:7)',quatmultiply([0 hw(1:3)'],quatconj(x(4:7)')))';
hint1r = quatmultiply(x(4:7)',quatmultiply([0 hw(4:6)'],quatconj(x(4:7)')))';
hint2  = quatmultiply(x(4:7)',quatmultiply([0 hw(7:9)'],quatconj(x(4:7)')))';
hint2r = quatmultiply(x(4:7)',quatmultiply([0 hw(10:12)'],quatconj(x(4:7)')))';
hint3  = quatmultiply(x(4:7)',quatmultiply([0 hw(13:15)'],quatconj(x(4:7)')))';
hint3r = quatmultiply(x(4:7)',quatmultiply([0 hw(16:18)'],quatconj(x(4:7)')))';
hint4  = quatmultiply(x(4:7)',quatmultiply([0 hw(19:21)'],quatconj(x(4:7)')))';
hint4r = quatmultiply(x(4:7)',quatmultiply([0 hw(22:24)'],quatconj(x(4:7)')))';


h_int = [hint1(2:4);
        hint1r(2:4);
        hint2(2:4);
        hint2r(2:4);
        hint3(2:4);
        hint3r(2:4);
        hint4(2:4);
        hint4r(2:4)];
